simulink model "FOCAL_MIMO_4x4_IndependentSISO_mdl_r2023b"  (R2023b)
settings: Solver=VariableStepAuto  StartTime=0.0  StopTime=10.0  RelTol=1e-3
values from neighbouring files (symbols this model uses):
  P0 = TF    [Copy_of_FOCAL_MIMO_4x4_IndependentSISO_Simulink_Linearization.m]    (also in FOCAL_MIMO_4x4_IndependentSISO_Simulink_Linearization.m = tf( P0 ))
settings Model: Creator=mohammadodeh  LastModifiedBy=mohammadodeh

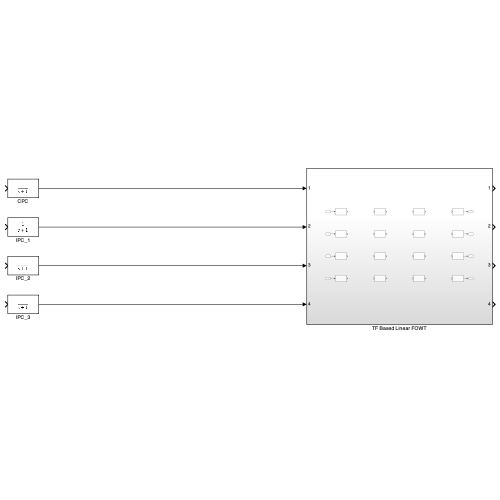
[thumbnail: Simulink's stored preview of the top-level diagram]
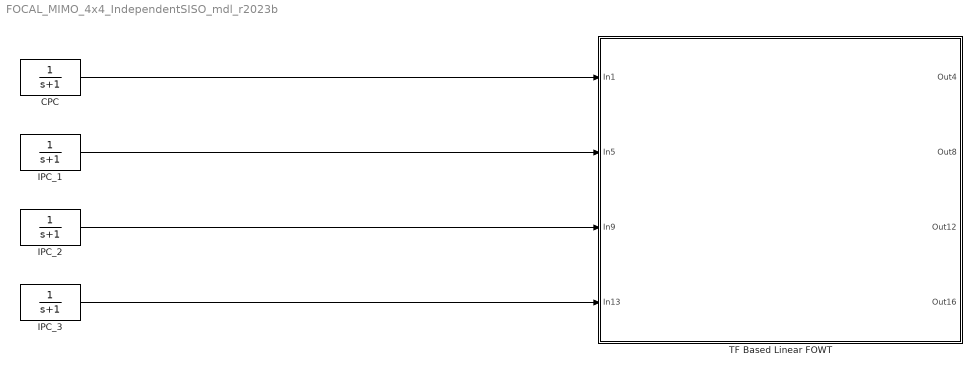
== system FOCAL_MIMO_4x4_IndependentSISO_mdl_r2023b ==
  CPC : TransferFcn  Denominator=[1 1]
  IPC_1 : TransferFcn  Denominator=[1 1]
  IPC_2 : TransferFcn  Denominator=[1 1]
  IPC_3 : TransferFcn  Denominator=[1 1]
  TF Based Linear FOWT : Subsystem
  wires:
  IPC_2/1 -> TF Based Linear FOWT/3(In9)
  IPC_1/1 -> TF Based Linear FOWT/2(In5)
  CPC/1 -> TF Based Linear FOWT/1(In1)
  IPC_3/1 -> TF Based Linear FOWT/4(In13)

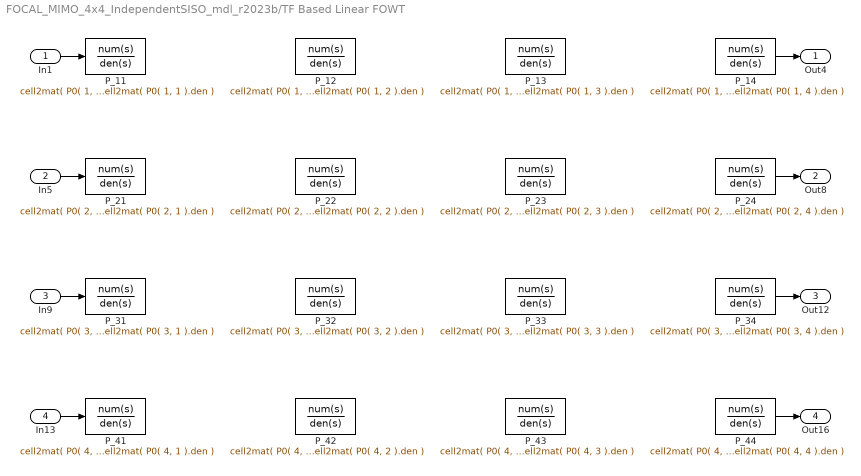
== system FOCAL_MIMO_4x4_IndependentSISO_mdl_r2023b/TF Based Linear FOWT ==
  In1 : Inport
  In5 : Inport  Port=2
  In9 : Inport  Port=3
  In13 : Inport  Port=4
  P_11 : TransferFcn  Numerator=cell2mat( P0( 1, 1 ).num )  Denominator=cell2mat( P0( 1, 1 ).den )
  P_12 : TransferFcn  Numerator=cell2mat( P0( 1, 2 ).num )  Denominator=cell2mat( P0( 1, 2 ).den )
  P_13 : TransferFcn  Numerator=cell2mat( P0( 1, 3 ).num )  Denominator=cell2mat( P0( 1, 3 ).den )
  P_14 : TransferFcn  Numerator=cell2mat( P0( 1, 4 ).num )  Denominator=cell2mat( P0( 1, 4 ).den )
  P_21 : TransferFcn  Numerator=cell2mat( P0( 2, 1 ).num )  Denominator=cell2mat( P0( 2, 1 ).den )
  P_22 : TransferFcn  Numerator=cell2mat( P0( 2, 2 ).num )  Denominator=cell2mat( P0( 2, 2 ).den )
  P_23 : TransferFcn  Numerator=cell2mat( P0( 2, 3 ).num )  Denominator=cell2mat( P0( 2, 3 ).den )
  P_24 : TransferFcn  Numerator=cell2mat( P0( 2, 4 ).num )  Denominator=cell2mat( P0( 2, 4 ).den )
  P_31 : TransferFcn  Numerator=cell2mat( P0( 3, 1 ).num )  Denominator=cell2mat( P0( 3, 1 ).den )
  P_32 : TransferFcn  Numerator=cell2mat( P0( 3, 2 ).num )  Denominator=cell2mat( P0( 3, 2 ).den )
  P_33 : TransferFcn  Numerator=cell2mat( P0( 3, 3 ).num )  Denominator=cell2mat( P0( 3, 3 ).den )
  P_34 : TransferFcn  Numerator=cell2mat( P0( 3, 4 ).num )  Denominator=cell2mat( P0( 3, 4 ).den )
  P_41 : TransferFcn  Numerator=cell2mat( P0( 4, 1 ).num )  Denominator=cell2mat( P0( 4, 1 ).den )
  P_42 : TransferFcn  Numerator=cell2mat( P0( 4, 2 ).num )  Denominator=cell2mat( P0( 4, 2 ).den )
  P_43 : TransferFcn  Numerator=cell2mat( P0( 4, 3 ).num )  Denominator=cell2mat( P0( 4, 3 ).den )
  P_44 : TransferFcn  Numerator=cell2mat( P0( 4, 4 ).num )  Denominator=cell2mat( P0( 4, 4 ).den )
  Out4 : Outport
  Out8 : Outport  Port=2
  Out12 : Outport  Port=3
  Out16 : Outport  Port=4
  wires:
  P_34/1 -> Out12/1
  P_14/1 -> Out4/1
  P_44/1 -> Out16/1
  P_24/1 -> Out8/1
  In5/1 -> P_21/1
  In9/1 -> P_31/1
  In13/1 -> P_41/1
  In1/1 -> P_11/1
